simulink model "CMG_Testbed"  (R2024b)
settings: Solver=FixedStepAuto  StartTime=0.0  StopTime=inf  RelTol=1e-3  EnableMultiTasking=on
values from neighbouring files (symbols this model uses):
  gamma1_initial = deg2rad(0)    [CMG_Statespace.m]
  gamma2_initial = deg2rad(0)    [CMG_Statespace.m]
  p1 = linspace(gamma1_min,gamma1_max,10)    [CMG_Statespace.m]
  p2 = linspace(gamma2_min,gamma2_max,10)    [CMG_Statespace.m]
undefined symbols (not defined in the file or in its folder): K1, K2, K3, K4
libraries: simulink_extras x5, arduinolib x4, cstblocks x1, arduinosensorlib x1, sldrtlib x1
settings Model: ExtModeTrigDuration=2  Creator=lanhi  LastModifiedBy=lanhi
settings SolverCC: AutoInsertRateTranBlk=on
settings OptimizationCC: EnhancedBackFolding=on  PassReuseOutputArgsThreshold=0  MaxStackSize=64  OptimizeBlockOrder=speed  DifferentSizesBufferReuse=on  OptimizationCustomize=off
settings DebuggingCC: ParameterTunabilityLossMsg=error
settings HardwareCC: ProdBitPerPointer=32  ProdBitPerSizeT=32  ProdBitPerPtrDiffT=32  ProdLargestAtomicInteger=Long  ProdLargestAtomicFloat=Double  ProdWordSize=32  ProdHWDeviceType=ARM Compatible->ARM Cortex  UseEmbeddedCoderFeatures=off  UseSimulinkCoderFeatures=off
settings SFSimCC: MATLABDynamicMemAlloc=off
settings RTWCC: Description=Embedded Coder  SystemTargetFile=ert.tlc  HardwareBoard=ESP32-WROOM(Arduino Compatible)  TLCOptions="-aInlineSetEventsForThisBaseRateFcn=TLC_FALSE -aSuppressMultiTaskScheduler=TLC_FALSE    -aRateBasedStepFcn=0"  TemplateMakefile=ert_default_tmf  Toolchain=ESP32  BuildConfiguration=Faster Runs
settings CodeAppCC: ForceParamTrailComments=on  OperatorAnnotations=on  MangleLength=10
settings ERTTargetCC: ERTCustomFileBanners=off  SupportContinuousTime=on  SupportNonInlinedSFcns=on  RemoveResetFunc=off  SupportVariableSizeSignals=on  ModelStepFunctionPrototypeControlCompliant=off  ExtModeTransport=3  ExtModeStaticAlloc=on  ExtModeAutomaticAllocSize=off  ExtModeStaticAllocSize=65536  ExtModeMexFile=ext_xcp  ExtModeIntrfLevel=Level2 - Open  InlinedParameterPlacement=Hierarchical  DynamicArrayContainerType=coder::array

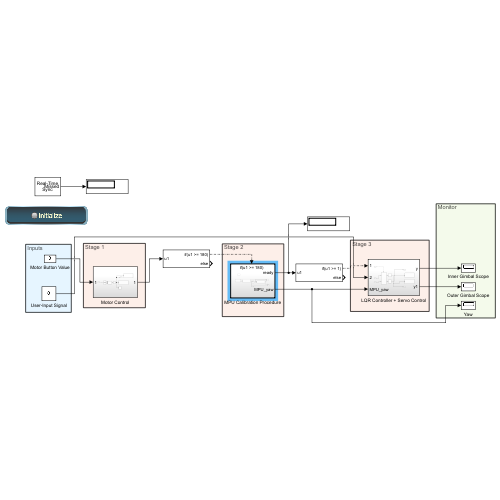
[thumbnail: Simulink's stored preview of the top-level diagram]
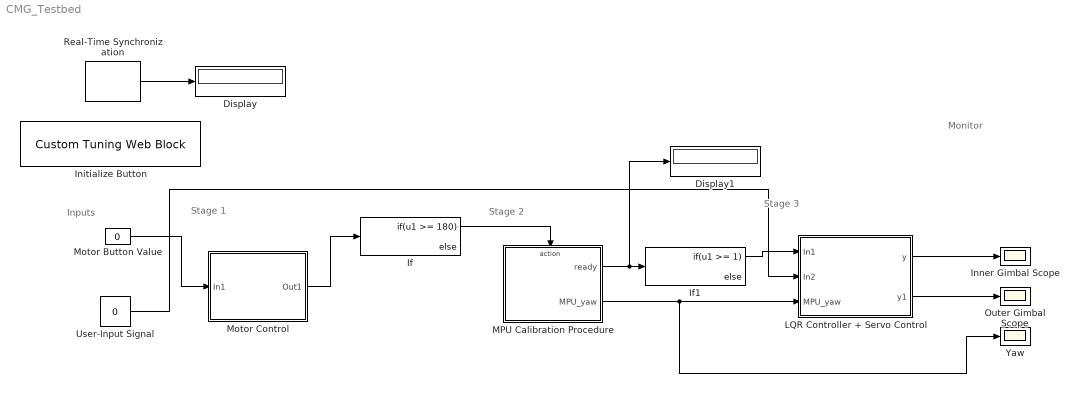
== system CMG_Testbed ==
  note: Inputs
  note: Monitor
  note: Stage 3
  note: Stage 2
  note: Stage 1
  Display : Display
  Display1 : Display
  If : If  IfExpression=u1 >= 180
  If1 : If  IfExpression=u1 >= 1
  Initialize Button : CustomTuningWebBlock  LabelPosition=Hide  ShowInitialText=on  Configuration="{\"components\":[{\"name\":\"BackgroundImageComponent\",\"settings\":{\"image\":{\"size\":[0,0],\"src\":\"default\",\"srcOrientation\":\"horizontal\"},\"position\":[0,0,1,1],\"scaleMode\":\"0\"}},{\"name\":\"ButtonStateComponent\",\"settings\":{\"buttonType\":\"latch\",\"clickFcn\":\"\",\"image\":{\"size\":[180,45],\"srcOrientation\":\"Right\"},\"latched\":false,\"offValue\":null,\"onValue\":\"1\",\"position\":[0,0,1,1],\"pressDelay\":\"500\",\"pressFcn\":\"\",\"repeatInterval\":\"0\",\"states\":[{\"horizontalAlignment\":\"center\",\"image\":{\"position\":[0.04444444444444445,0.005555555555555536,0.9888888888888889,0.9111111111111111],\"size\":[0.9888888888888889,0.9111111111111111],\"src\":\"data:image\\/svg+xml;base64,PHN2ZyB4bWxucz0iaHR0cDovL3d3dy53My5vcmcvMjAwMC9zdmciIHhtbG5zOnhsaW5rPSJodHRwOi8vd3d3LnczLm9yZy8xOTk5L3hsaW5rIiB2aWV3Qm94PSIwIDAgMTc3LjI1IDQwLjg4Ij48ZGVmcz48c3R5bGU+LmNscy0xe2ZpbGw6dXJsKCNyYWRpYWwtZ3JhZGllbnQpO30uY2xzLTJ7ZmlsbDp1cmwoI2xpbmVhci1ncmFkaWVudCk7fS5jbHMtM3tmaWxsOnVybCgjbGluZWFyLWdyYWRpZW50LTIpO308L3N0eWxlPjxyYWRpYWxHcmFkaWVudCBpZD0icmFkaWFsLWdyYWRpZW50IiBjeD0iOTAuMDkiIGN5PSIyMi42NiIgcj0i ...(+2212 chars)\",\"srcOrientation\":\"Right\"},\"label\":{\"color\":[1,1,0.78,1],\"icon\":{\"size\":[1.2903018954534844,1.2096580269876416],\"src\":\"data:image\\/svg+xml;base64,PHN2ZyBpZD0iT2ZmIiB4bWxucz0iaHR0cDovL3d3dy53My5vcmcvMjAwMC9zdmciIHhtbG5zOnhsaW5rPSJodHRwOi8vd3d3LnczLm9yZy8xOTk5L3hsaW5rIiB2aWV3Qm94PSIwIDAgNTAgNTAiPjxkZWZzPjxzdHlsZT4uY2xzLTF7ZmlsbDojN2Y4MDgwO3N0cm9rZTojMjcyNjI2O3N0cm9rZS1taXRlcmxpbWl0OjEwO3N0cm9rZS13aWR0aDozcHg7fS5jbHMtMntmaWxsOnVybCgjbGluZWFyLWdyYWRpZW50KTt9PC9zdHlsZT48bGluZWFyR3JhZGllbnQgaWQ9ImxpbmVhci1ncmFkaWVudCIgeDE9IjI1IiB5MT0iOSIgeDI9IjI1IiB5Mj0iMzciIGdyYWRpZW50VW5pdHM9InVzZXJTcGFjZU9uVXNlIj48c3RvcCBvZmZzZXQ9IjAiIHN0b3AtY29sb3I9IiNmZmYiIHN0b3Atb3BhY2l0eT0iMC43NSIvPjxzdG9wIG9mZnNldD0iMSIgc3RvcC1jb2xvcj0iI2ZmZiIgc3RvcC1vcGFjaXR5PSIwIi8+PC9saW5lYXJHcmFkaWVudD48L2RlZnM+PGNpcmNsZSBjbGFzcz0iY2xzLTEiIGN4PSIyNSIgY3k9IjI1IiByPSIyMCIvPjxjaXJjbGUgY2xhc3M9ImNscy0yIiBjeD0iMjUiIGN5PSIyMyIgcj0iMTQiLz48L3N2Zz4=\",\"srcOrientation\":\"Right\"},\"iconOffset\":0,\"iconPlacement\":\"left\",\"opacity\":1,\"show\":true,\"text\":{\"content\":\"Initialize\",\"font\":\"Helvetica\"}},\"labelOffset\":[0,0],\"verticalAlignment\":\"middle\"},{\"horizontalAlignment\":\"center\",\"image\":{\"position\":[0.04444444444444445,0.005555555555555536,0.9888888888888889,0.9111111111111111],\"size\":[0.9888888888888889,0.9111111111111111],\"src\":\"data:image\\/svg+xml;base64,PHN2ZyB4bWxucz0iaHR0cDovL3d3dy53My5vcmcvMjAwMC9zdmciIHhtbG5zOnhsaW5rPSJodHRwOi8vd3d3LnczLm9yZy8xOTk5L3hsaW5rIiB2aWV3Qm94PSIwIDAgMTc3LjI1IDQwLjg4Ij48ZGVmcz48c3R5bGU+LmNscy0xe2ZpbGw6dXJsKCNyYWRpYWwtZ3JhZGllbnQpO30uY2xzLTJ7ZmlsbDp1cmwoI2xpbmVhci1ncmFkaWVudCk7fS5jbHMtM3tmaWxsOnVybCgjbGluZWFyLWdyYWRpZW50LTIpO308L3N0eWxlPjxyYWRpYWxHcmFkaWVudCBpZD0icmFkaWFsLWdyYWRpZW50IiBjeD0iOTAuMDkiIGN5PSIyMi42NiIgcj0i ...(+2216 chars)\",\"srcOrientation\":\"Right\"},\"label\":{\"color\":[1,1,0.78,1],\"icon\":{\"size\":[1.2903018954534844,1.2096580269876416],\"src\":\"data:image\\/svg+xml;base64,PHN2ZyB4bWxucz0iaHR0cDovL3d3dy53My5vcmcvMjAwMC9zdmciIHhtbG5zOnhsaW5rPSJodHRwOi8vd3d3LnczLm9yZy8xOTk5L3hsaW5rIiB2aWV3Qm94PSIwIDAgNTAgNTAiPjxkZWZzPjxzdHlsZT4uY2xzLTF7ZmlsbDojNmFiZDQ1O3N0cm9rZTojMjcyNjI2O3N0cm9rZS1taXRlcmxpbWl0OjEwO3N0cm9rZS13aWR0aDozcHg7fS5jbHMtMntmaWxsOnVybCgjbGluZWFyLWdyYWRpZW50KTt9PC9zdHlsZT48bGluZWFyR3JhZGllbnQgaWQ9ImxpbmVhci1ncmFkaWVudCIgeDE9IjI1IiB5MT0iOSIgeDI9IjI1IiB5Mj0iMzciIGdyYWRpZW50VW5pdHM9InVzZXJTcGFjZU9uVXNlIj48c3RvcCBvZmZzZXQ9IjAiIHN0b3AtY29sb3I9IiNmZmYiIHN0b3Atb3BhY2l0eT0iMC43NSIvPjxzdG9wIG9mZnNldD0iMSIgc3RvcC1jb2xvcj0iI2ZmZiIgc3RvcC1vcGFjaXR5PSIwIi8+PC9saW5lYXJHcmFkaWVudD48L2RlZnM+PGcgaWQ9Ik9uIj48Y2lyY2xlIGNsYXNzPSJjbHMtMSIgY3g9IjI1IiBjeT0iMjUiIHI9IjIwIi8+PGNpcmNsZSBjbGFzcz0iY2xzLTIiIGN4PSIyNSIgY3k9IjIzIiByPSIxNCIvPjwvZz48L3N2Zz4=\",\"srcOrientation\":\"Right\"},\"iconOffset\":0,\"iconPlacement\":\"left\",\"opacity\":1,\"show\":true,\"text\":{\"content\":\"Initialize\",\"font\":\"Helvetica\"}},\"labelOffset\":[0.025,0],\"verticalAlignment\":\"middle\"},{\"horizontalAlignment\":\"center\",\"image\":{\"position\":[0.04444444444444445,0.005555555555555536,0.9888888888888889,0.9111111111111111],\"size\":[0.9888888888888889,0.9111111111111111],\"src\":\"data:image\\/svg+xml;base64,PHN2ZyB4bWxucz0iaHR0cDovL3d3dy53My5vcmcvMjAwMC9zdmciIHhtbG5zOnhsaW5rPSJodHRwOi8vd3d3LnczLm9yZy8xOTk5L3hsaW5rIiB2aWV3Qm94PSIwIDAgMTc3LjI1IDQwLjg4Ij48ZGVmcz48c3R5bGU+LmNscy0xe2ZpbGw6dXJsKCNyYWRpYWwtZ3JhZGllbnQpO30uY2xzLTJ7ZmlsbDp1cmwoI2xpbmVhci1ncmFkaWVudCk7fS5jbHMtM3tmaWxsOnVybCgjbGluZWFyLWdyYWRpZW50LTIpO308L3N0eWxlPjxyYWRpYWxHcmFkaWVudCBpZD0icmFkaWFsLWdyYWRpZW50IiBjeD0iOTAuMDkiIGN5PSIyMi42NiIgcj0i ...(+2212 chars)\",\"srcOrientation\":\"Right\"},\"label\":{\"color\":[1,1,0.78,1],\"icon\":{\"size\":[1.2903018954534844,1.2096580269876416],\"src\":\"data:image\\/svg+xml;base64,PHN2ZyB4bWxucz0iaHR0cDovL3d3dy53My5vcmcvMjAwMC9zdmciIHhtbG5zOnhsaW5rPSJodHRwOi8vd3d3LnczLm9yZy8xOTk5L3hsaW5rIiB2aWV3Qm94PSIwIDAgNTAgNTAiPjxkZWZzPjxzdHlsZT4uY2xzLTF7ZmlsbDojNmFiZDQ1O3N0cm9rZTojMjcyNjI2O3N0cm9rZS1taXRlcmxpbWl0OjEwO3N0cm9rZS13aWR0aDozcHg7fS5jbHMtMntmaWxsOnVybCgjbGluZWFyLWdyYWRpZW50KTt9PC9zdHlsZT48bGluZWFyR3JhZGllbnQgaWQ9ImxpbmVhci1ncmFkaWVudCIgeDE9IjI1IiB5MT0iOSIgeDI9IjI1IiB5Mj0iMzciIGdyYWRpZW50VW5pdHM9InVzZXJTcGFjZU9uVXNlIj48c3RvcCBvZmZzZXQ9IjAiIHN0b3AtY29sb3I9IiNmZmYiIHN0b3Atb3BhY2l0eT0iMC43NSIvPjxzdG9wIG9mZnNldD0iMSIgc3RvcC1jb2xvcj0iI2ZmZiIgc3RvcC1vcGFjaXR5PSIwIi8+PC9saW5lYXJHcmFkaWVudD48L2RlZnM+PGcgaWQ9Ik9uIj48Y2lyY2xlIGNsYXNzPSJjbHMtMSIgY3g9IjI1IiBjeT0iMjUiIHI9IjIwIi8+PGNpcmNsZSBjbGFzcz0iY2xzLTIiIGN4PSIyNSIgY3k9IjIzIiByPSIxNCIvPjwvZz48L3N2Zz4=\",\"srcOrientation\":\"Right\"},\"iconOffset\":0,\"iconPlacement\":\"left\",\"opacity\":1,\"show\":true,\"text\":{\"content\":\"Initialize\",\"font\":\"Helvetica\"}},\"labelOffset\":[0,0],\"verticalAlignment\":\"middle\"},{\"horizontalAlignment\":\"center\",\"image\":{\"position\":[0.04444444444444445,0.005555555555555536,0.9888888888888889,0.9111111111111111],\"size\":[0.9888888888888889,0.9111111111111111],\"src\":\"data:image\\/svg+xml;base64,PHN2ZyB4bWxucz0iaHR0cDovL3d3dy53My5vcmcvMjAwMC9zdmciIHhtbG5zOnhsaW5rPSJodHRwOi8vd3d3LnczLm9yZy8xOTk5L3hsaW5rIiB2aWV3Qm94PSIwIDAgMTc3LjI1IDQwLjg4Ij48ZGVmcz48c3R5bGU+LmNscy0xe2ZpbGw6dXJsKCNyYWRpYWwtZ3JhZGllbnQpO30uY2xzLTJ7ZmlsbDp1cmwoI2xpbmVhci1ncmFkaWVudCk7fS5jbHMtM3tmaWxsOnVybCgjbGluZWFyLWdyYWRpZW50LTIpO308L3N0eWxlPjxyYWRpYWxHcmFkaWVudCBpZD0icmFkaWFsLWdyYWRpZW50IiBjeD0iOTAuMDkiIGN5PSIyMi42NiIgcj0i ...(+2216 chars)\",\"srcOrientation\":\"Right\"},\"label\":{\"color\":[1,1,0.78,1],\"icon\":{\"size\":[1.2903018954534844,1.2096580269876416],\"src\":\"data:image\\/svg+xml;base64,PHN2ZyBpZD0iT2ZmIiB4bWxucz0iaHR0cDovL3d3dy53My5vcmcvMjAwMC9zdmciIHhtbG5zOnhsaW5rPSJodHRwOi8vd3d3LnczLm9yZy8xOTk5L3hsaW5rIiB2aWV3Qm94PSIwIDAgNTAgNTAiPjxkZWZzPjxzdHlsZT4uY2xzLTF7ZmlsbDojN2Y4MDgwO3N0cm9rZTojMjcyNjI2O3N0cm9rZS1taXRlcmxpbWl0OjEwO3N0cm9rZS13aWR0aDozcHg7fS5jbHMtMntmaWxsOnVybCgjbGluZWFyLWdyYWRpZW50KTt9PC9zdHlsZT48bGluZWFyR3JhZGllbnQgaWQ9ImxpbmVhci1ncmFkaWVudCIgeDE9IjI1IiB5MT0iOSIgeDI9IjI1IiB5Mj0iMzciIGdyYWRpZW50VW5pdHM9InVzZXJTcGFjZU9uVXNlIj48c3RvcCBvZmZzZXQ9IjAiIHN0b3AtY29sb3I9IiNmZmYiIHN0b3Atb3BhY2l0eT0iMC43NSIvPjxzdG9wIG9mZnNldD0iMSIgc3RvcC1jb2xvcj0iI2ZmZiIgc3RvcC1vcGFjaXR5PSIwIi8+PC9saW5lYXJHcmFkaWVudD48L2RlZnM+PGNpcmNsZSBjbGFzcz0iY2xzLTEiIGN4PSIyNSIgY3k9IjI1IiByPSIyMCIvPjxjaXJjbGUgY2xhc3M9ImNscy0yIiBjeD0iMjUiIGN5PSIyMyIgcj0iMTQiLz48L3N2Zz4=\",\"srcOrientation\":\"Right\"},\"iconOffset\":0,\"iconPlacement\":\"left\",\"opacity\":1,\"show\":true,\"text\":{\"content\":\"Initialize\",\"font\":\"Helvetica\"}},\"labelOffset\":[0.025,0],\"verticalAlignment\":\"middle\"}]}},{\"name\":\"ForegroundImageComponent\",\"settings\":{\"image\":{\"size\":[0,0],\"src\":\"default\",\"srcOrientation\":\"horizontal\"},\"isForeground\":1,\"position\":[0,0,1,1],\"scaleMode\":\"0\"}}],\"settings\":{\"BindingType\":\"param\",\"aspectRatio\":3.7777777777777777,\"backgroundColor\":[0,0,0,\"1\"],\"backgroundOffset\":0,\"backgroundOpacity\":1,\"fixedAspectRatio\":\"on\",\"foregroundColor\":[252,252,196],\"showBackgroundColor\":false,\"variant\":\"push\",\"version\":\"R2024b\"},\"type\":\"Button\"}"
  Inner Gimbal Scope : Scope
  LQR Controller + Servo Control : Subsystem
  MPU Calibration Procedure : Subsystem  TreatAsAtomicUnit=on
  Motor Button Value : Constant  Value=0
  Motor Control : Subsystem
  Outer Gimbal Scope : Scope
  Real-Time Synchronization : sldrtlib/Real-Time Synchronization  SampleTime=0.1  MaxMissedTicks=500  ShowMissedTicks=on  YieldWhenWaiting=off
  User-Input Signal : Constant  Value=0
  Yaw : Scope
  wires:
  If/1 -> MPU Calibration Procedure/Action
  MPU Calibration Procedure/1(ready) -> Display1/1, If1/1
  Motor Button Value/1 -> Motor Control/1(In1)
  Motor Control/1(Out1) -> If/1
  If1/1 -> LQR Controller + Servo Control/1(In1)
  User-Input Signal/1 -> LQR Controller + Servo Control/2(In2)
  LQR Controller + Servo Control/1(y) -> Inner Gimbal Scope/1
  LQR Controller + Servo Control/2(y1) -> Outer Gimbal Scope/1
  MPU Calibration Procedure/2(MPU_yaw) -> LQR Controller + Servo Control/3(MPU_yaw), Yaw/1
  Real-Time Synchronization/1 -> Display/1

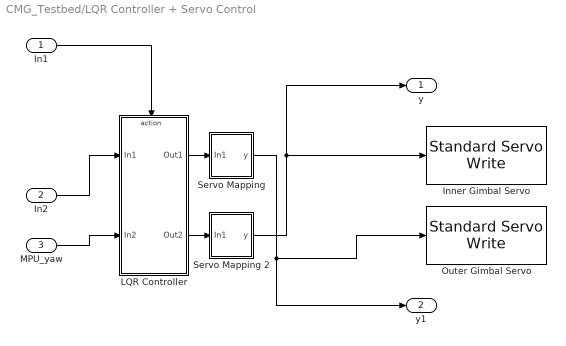
== system CMG_Testbed/LQR Controller + Servo Control ==
  In1 : Inport
  In2 : Inport  Port=2
  MPU_yaw : Inport  Port=3
  Inner Gimbal Servo : arduinolib/Standard Servo Write  pinNumber=4  ServoIndex=0  blockPlatform=ARDUINO
  LQR Controller : Subsystem  TreatAsAtomicUnit=on
  Outer Gimbal Servo : arduinolib/Standard Servo Write  pinNumber=5  ServoIndex=1  blockPlatform=ARDUINO
  Servo Mapping : Subsystem
  Servo Mapping 2 : Subsystem
  y : Outport
  y1 : Outport  Port=2
  wires:
  LQR Controller/2(Out2) -> Servo Mapping 2/1(In1)
  LQR Controller/1(Out1) -> Servo Mapping/1(In1)
  In2/1 -> LQR Controller/1(In1)
  In1/1 -> LQR Controller/Action
  MPU_yaw/1 -> LQR Controller/2(In2)
  Servo Mapping/1(y) -> Outer Gimbal Servo/1, y1/1
  Servo Mapping 2/1(y) -> Inner Gimbal Servo/1, y/1

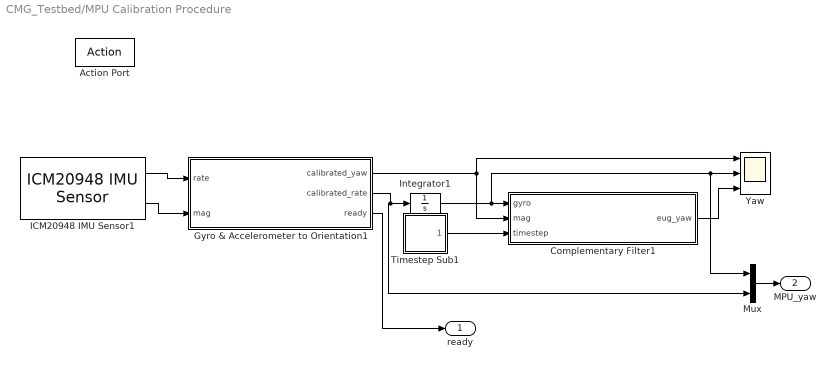
== system CMG_Testbed/MPU Calibration Procedure ==
  Action Port : ActionPort  ActionPortLabel=if(u1 >= 180)
  Complementary Filter1 : MATLAB Function  TreatAsAtomicUnit=on
  Gyro & Accelerometer to Orientation1 : MATLAB Function  TreatAsAtomicUnit=on
  ICM20948 IMU Sensor1 : arduinosensorlib/ICM20948 IMU Sensor  I2CModule=0  I2CAddress=0x69  BitRate=1000000  EnableDRDY=on  InterruptType=Active high  IsActiveAccel=off  IsActiveGyro=on  IsActiveMag=on  IsActiveTemp=off  IsActiveStatus=off  IsActiveTimeStamp=off  AccelerometerRange=+/-2g  AccelerometerODR=1125  AccelerometerBW=23.9 Hz  GyroscopeRange=+/-250 dps  GyroscopeODR=1125  GyroscopeBW=23.9 Hz  MagnetometerODR=100 Hz  TemperatureBW=34.1 Hz  DataType=double  spf=1  SampleTime=-1  QueueSizeFactor=1
  Integrator1 : Integrator
  Mux : Mux  Inputs=2
  Timestep Sub1 : Subsystem
  Yaw : Scope  NumInputPorts=3
  ready : Outport
  MPU_yaw : Outport  Port=2
  wires:
  Timestep Sub1/1(timestep) -> Complementary Filter1/3(timestep)
  Gyro & Accelerometer to Orientation1/1(calibrated_yaw) -> Complementary Filter1/2(mag), Yaw/1
  Integrator1/1 -> Mux/1, Yaw/2, Complementary Filter1/1(gyro)
  ICM20948 IMU Sensor1/1 -> Gyro & Accelerometer to Orientation1/1(rate)
  Complementary Filter1/1(eug_yaw) -> Yaw/3
  ICM20948 IMU Sensor1/2 -> Gyro & Accelerometer to Orientation1/2(mag)
  Gyro & Accelerometer to Orientation1/2(calibrated_rate) -> Integrator1/1, Mux/2
  Gyro & Accelerometer to Orientation1/3(ready) -> ready/1
  Mux/1 -> MPU_yaw/1

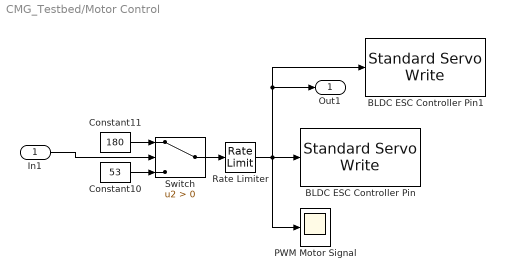
== system CMG_Testbed/Motor Control ==
  In1 : Inport
  BLDC ESC Controller Pin : arduinolib/Standard Servo Write  pinNumber=18  ServoIndex=2  blockPlatform=ARDUINO
  BLDC ESC Controller Pin1 : arduinolib/Standard Servo Write  pinNumber=19  ServoIndex=3  blockPlatform=ARDUINO
  Constant10 : Constant  Value=53
  Constant11 : Constant  Value=180
  PWM Motor Signal : Scope
  Rate Limiter : RateLimiter  RisingSlewLimit=25  FallingSlewLimit=-25  SampleTimeMode=inherited  InitialCondition=53
  Switch : Switch  Criteria=u2 > Threshold  SaturateOnIntegerOverflow=off  InputSameDT=off
  Out1 : Outport
  wires:
  Switch/1 -> Rate Limiter/1
  In1/1 -> Switch/2
  Constant10/1 -> Switch/3
  Rate Limiter/1 -> BLDC ESC Controller Pin/1, BLDC ESC Controller Pin1/1, Out1/1, PWM Motor Signal/1
  Constant11/1 -> Switch/1

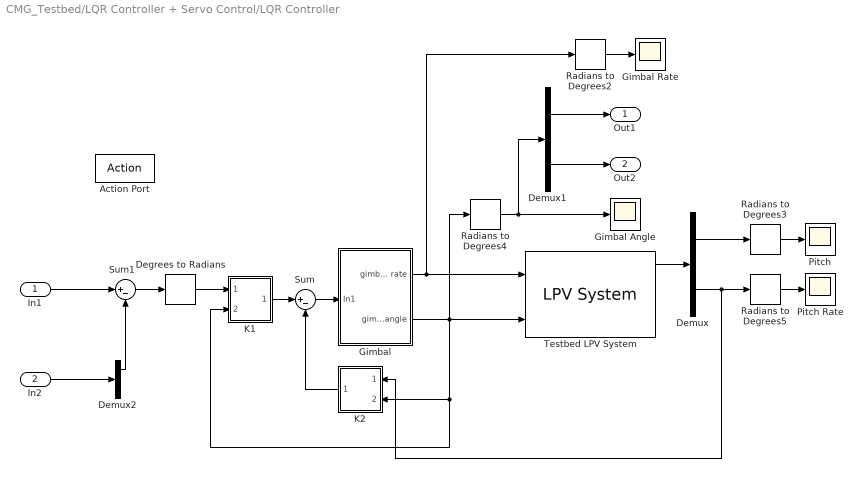
== system CMG_Testbed/LQR Controller + Servo Control/LQR Controller ==
  In1 : Inport
  In2 : Inport  Port=2
  Action Port : ActionPort  ActionPortLabel=if(u1 >= 1)
  Degrees to Radians : simulink_extras/Transformations/Degrees to Radians
  Demux : Demux  Outputs=2
  Demux1 : Demux  Outputs=2
  Demux2 : Demux  Outputs=2
  Gimbal : Subsystem
  Gimbal Angle : Scope
  Gimbal Rate : Scope
  K1 : Subsystem
  K2 : Subsystem
  Pitch : Scope
  Pitch Rate : Scope
  Radians to Degrees{2..5} (4 alike) : simulink_extras/Transformations/Radians to Degrees
  Sum : Sum  Inputs=|+-
  Sum1 : Sum  Inputs=|+-
  Testbed LPV System : cstblocks/Linear Parameter Varying/LPV System  sys=ICs  InitialConditionSource=internal  InitialCondition=[deg2rad(0),0]  opSpecOption=Specify offsets as double arrays  uOffset=0  yOffset=0  xOffset=0  opEquilOption=on  dxOffset=0  AFixed=false  BFixed=false  CFixed=false  DFixed=false  uDelayFixed=false  yDelayFixed=false  iDelayFixed=false  sysFixedOption=First model in state-space array  sysFixed=[]  IMethod=Linear  EMethod=Clip  IndexSearch=Binary search  IndexBegin=on  OutputX=on  OutputXdot=on  OutputLTI=on  OutputOP=on  DataType=double  InitBufferSize=1024  FixedBuffer=off  SimMode=Interpreted execution  Offset=struct
  Out1 : Outport
  Out2 : Outport  Port=2
  wires:
  K2/1(Out1) -> Sum/2
  Demux/2 -> K2/1(In1), Radians to Degrees5/1
  Testbed LPV System/1 -> Demux/1
  Radians to Degrees2/1 -> Gimbal Rate/1
  Gimbal/1(gimbal ang rate) -> Testbed LPV System/1, Radians to Degrees2/1
  K1/1(Out1) -> Sum/1
  Sum/1 -> Gimbal/1(In1)
  Demux/1 -> Radians to Degrees3/1
  Radians to Degrees5/1 -> Pitch Rate/1
  Gimbal/2(gimbal angle) -> Testbed LPV System/2, Radians to Degrees4/1, K1/2(In2), K2/2(In2)
  Radians to Degrees3/1 -> Pitch/1
  Radians to Degrees4/1 -> Gimbal Angle/1, Demux1/1
  Demux1/1 -> Out1/1
  Demux1/2 -> Out2/1
  In1/1 -> Sum1/1
  Sum1/1 -> Degrees to Radians/1
  Degrees to Radians/1 -> K1/1(In1)
  In2/1 -> Demux2/1
  Demux2/1 -> Sum1/2

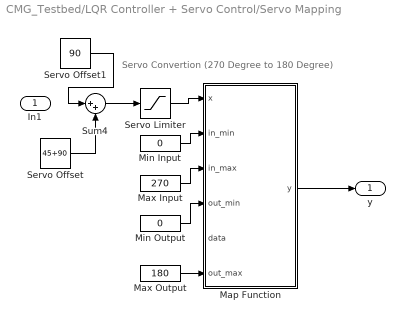
== system CMG_Testbed/LQR Controller + Servo Control/Servo Mapping ==
  note: Servo Convertion (270 Degree to 180 Degree)
  In1 : Inport
  Map Function : MATLAB Function  TreatAsAtomicUnit=on
  Max Input : Constant  Value=270
  Max Output : Constant  Value=180
  Min Input : Constant  Value=0
  Min Output : Constant  Value=0
  Servo Limiter : Saturate  UpperLimit=225  LowerLimit=45
  Servo Offset : Constant  Value=45+90
  Servo Offset1 : Constant  Value=90
  Sum4 : Sum  Inputs=|++
  y : Outport
  wires:
  Max Input/1 -> Map Function/3(in_max)
  Min Output/1 -> Map Function/4(out_min)
  Min Input/1 -> Map Function/2(in_min)
  Max Output/1 -> Map Function/6(out_max)
  Servo Limiter/1 -> Map Function/1(x)
  Sum4/1 -> Servo Limiter/1
  Servo Offset/1 -> Sum4/2
  Map Function/1(y) -> y/1
  Servo Offset1/1 -> Sum4/1

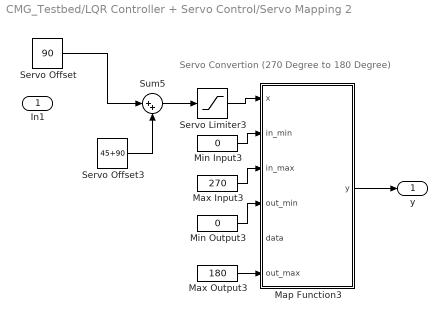
== system CMG_Testbed/LQR Controller + Servo Control/Servo Mapping 2 ==
  note: Servo Convertion (270 Degree to 180 Degree)
  In1 : Inport
  Map Function3 : MATLAB Function  TreatAsAtomicUnit=on
  Max Input3 : Constant  Value=270
  Max Output3 : Constant  Value=180
  Min Input3 : Constant  Value=0
  Min Output3 : Constant  Value=0
  Servo Limiter3 : Saturate  UpperLimit=225  LowerLimit=45
  Servo Offset : Constant  Value=90
  Servo Offset3 : Constant  Value=45+90
  Sum5 : Sum  Inputs=|++
  y : Outport
  wires:
  Min Output3/1 -> Map Function3/4(out_min)
  Min Input3/1 -> Map Function3/2(in_min)
  Sum5/1 -> Servo Limiter3/1
  Servo Limiter3/1 -> Map Function3/1(x)
  Map Function3/1(y) -> y/1
  Servo Offset3/1 -> Sum5/2
  Max Input3/1 -> Map Function3/3(in_max)
  Max Output3/1 -> Map Function3/6(out_max)
  Servo Offset/1 -> Sum5/1

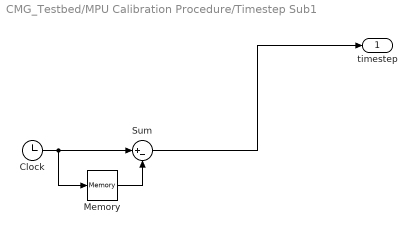
== system CMG_Testbed/MPU Calibration Procedure/Timestep Sub1 ==
  Clock : Clock
  Memory : Memory
  Sum : Sum  Inputs=|+-
  timestep : Outport
  wires:
  Memory/1 -> Sum/2
  Clock/1 -> Memory/1, Sum/1
  Sum/1 -> timestep/1

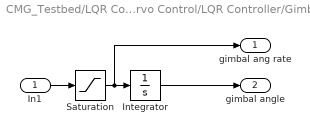
== system CMG_Testbed/LQR Controller + Servo Control/LQR Controller/Gimbal ==
  In1 : Inport
  Integrator : Integrator  InitialCondition=[gamma1_initial,gamma2_initial]
  Saturation : Saturate  UpperLimit=9.519977738135207  LowerLimit=-9.519977738135207
  gimbal ang rate : Outport
  gimbal angle : Outport  Port=2
  wires:
  Integrator/1 -> gimbal angle/1
  In1/1 -> Saturation/1
  Saturation/1 -> gimbal ang rate/1, Integrator/1

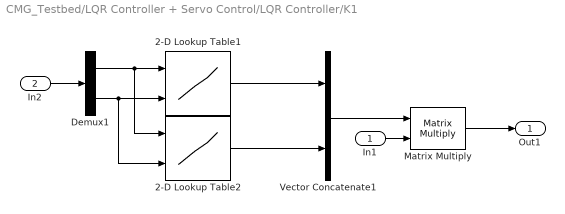
== system CMG_Testbed/LQR Controller + Servo Control/LQR Controller/K1 ==
  In1 : Inport
  In2 : Inport  Port=2
  2-D Lookup Table1 : Lookup_n-D  BreakpointsForDimension1=p1  BreakpointsForDimension2=p2  Table=K1  InternalRulePriority=Speed  RndMeth=Simplest
      settings: InputPortMap=u0,u1
  2-D Lookup Table2 : Lookup_n-D  BreakpointsForDimension1=p1  BreakpointsForDimension2=p2  Table=K3  InternalRulePriority=Speed  RndMeth=Simplest
      settings: InputPortMap=u0,u1
  Demux1 : Demux  Outputs=2
  Matrix Multiply : Product  Multiplication=Matrix(*)
  Vector Concatenate1 : Concatenate
  Out1 : Outport
  wires:
  Demux1/1 -> 2-D Lookup Table2/1, 2-D Lookup Table1/1
  Vector Concatenate1/1 -> Matrix Multiply/1
  2-D Lookup Table2/1 -> Vector Concatenate1/2
  Demux1/2 -> 2-D Lookup Table2/2, 2-D Lookup Table1/2
  2-D Lookup Table1/1 -> Vector Concatenate1/1
  In2/1 -> Demux1/1
  In1/1 -> Matrix Multiply/2
  Matrix Multiply/1 -> Out1/1

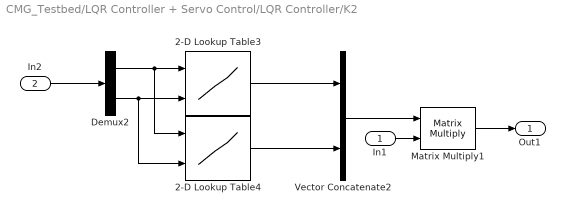
== system CMG_Testbed/LQR Controller + Servo Control/LQR Controller/K2 ==
  In1 : Inport
  In2 : Inport  Port=2
  2-D Lookup Table3 : Lookup_n-D  BreakpointsForDimension1=p1  BreakpointsForDimension2=p2  Table=K2  InternalRulePriority=Speed  RndMeth=Simplest
      settings: InputPortMap=u0,u1
  2-D Lookup Table4 : Lookup_n-D  BreakpointsForDimension1=p1  BreakpointsForDimension2=p2  Table=K4  InternalRulePriority=Speed  RndMeth=Simplest
      settings: InputPortMap=u0,u1
  Demux2 : Demux  Outputs=2
  Matrix Multiply1 : Product  Multiplication=Matrix(*)
  Vector Concatenate2 : Concatenate
  Out1 : Outport
  wires:
  Demux2/1 -> 2-D Lookup Table4/1, 2-D Lookup Table3/1
  Demux2/2 -> 2-D Lookup Table4/2, 2-D Lookup Table3/2
  2-D Lookup Table4/1 -> Vector Concatenate2/2
  2-D Lookup Table3/1 -> Vector Concatenate2/1
  Vector Concatenate2/1 -> Matrix Multiply1/1
  Matrix Multiply1/1 -> Out1/1
  In2/1 -> Demux2/1
  In1/1 -> Matrix Multiply1/2

== matlab function CMG_Testbed/MPU Calibration Procedure/Complementary Filter1 ==
  settings: updateMethod=DISCRETE
  data: gyro input; eug_yaw output; mag input; timestep input
function eug_yaw = CompFilter(gyro,mag,timestep)

persistent yaw;

if isempty(yaw), yaw = [0]; end


alpha = 0.70;

yaw = alpha*(gyro(1,1)*timestep + yaw) + (1-alpha)*(mag(1,1));

eug_yaw = yaw;





%function eug_angle = CompFilter(gyro,acc_angle,timestep)

%persistent angle_1; persistent angle_2; persistent angle_3;

%if isempty(angle_1), angle_1 = [0]; end
%if isempty(angle_2), angle_2 = [0]; end
%if isempty(angle_3), angle_3 = [0]; end

%alpha = 0.80;

%angle_1 = alpha*(gyro(1,1)*timestep + angle_1) + (1-alpha)*(acc_angle(1,1));
%angle_2 = alpha*(gyro(2,1)*timestep + angle_2) + (1-alpha)*(acc_angle(2,1));
%angle_3 = gyro(3,1)*timestep + angle_3;

%eug_angle = [angle_1,angle_2,angle_3];

== matlab function CMG_Testbed/LQR Controller + Servo Control/Servo Mapping/Map Function ==
  data: x input; y output; in_min input; in_max input; out_min input; data input; out_max input
function y = map(x,in_min,in_max,out_min,data, out_max)
    y = (x - in_min) * (out_max - out_min) / (in_max - in_min) + out_min;
end

== matlab function CMG_Testbed/LQR Controller + Servo Control/Servo Mapping 2/Map Function3 ==
  data: x input; y output; in_min input; in_max input; out_min input; data input; out_max input
function y = map(x,in_min,in_max,out_min,data, out_max)
    y = (x - in_min) * (out_max - out_min) / (in_max - in_min) + out_min;
end

== matlab function CMG_Testbed/MPU Calibration Procedure/Gyro & Accelerometer to Orientation1 ==
  settings: updateMethod=DISCRETE
  data: rate input; mag input; calibrated_yaw output; calibrated_rate output; ready output
function [calibrated_yaw,calibrated_rate,ready]= EularAngle(rate,mag)

% ---------------- [Tunable User Variables] ---------------- %

n = 30; % Max Cycles for Calibrating IMU/MPU data

% ---------------- [Function Counter] ---------------- %
persistent callCount loopcycle;

if isempty(loopcycle), loopcycle = 0; end               % If caibration is done, then loop cycle = 1

    if isempty(callCount)
        callCount = 0; % Initialize on first call
    end
    callCount = callCount + 1; % +1 for each time the function is called

% ---------------- [Function Counter] ---------------- %

A = [0.025257 , 0.000062 , -0.000096;
    0.000062 , 0.023110 , -0.000343;
    -0.000096 , -0.000343 , 0.024714];

B = [-27.385238 , 6.142666 , -33.779326];

cal_Mag = A* (mag - B)';

Mag_yaw = rad2deg(atan2(cal_Mag(2,1),cal_Mag(1,1)));

% ---------------- [Defining Persistent Variables] ---------------- %
persistent average_rate offset_rate cal_rate;

if isempty(average_rate), average_rate = [0;0;0]; end   % Average Gyro Rate
if isempty(offset_rate), offset_rate = [0;0;0]; end     % Gyro Offset
if isempty(cal_rate), cal_rate = [0;0;0]; end           % Calibrated Gyro Rate

if callCount < n
    average_rate = average_rate + rate';
else

    offset_rate = average_rate/n;
    cal_rate = rate' - offset_rate;
    loopcycle = 1;
end

% ---------------- [Return] ---------------- %

calibrated_rate = rad2deg(cal_rate(3,1));
calibrated_yaw = Mag_yaw;
ready = loopcycle;
